simulink model "GasExample_V4"  (R2025b)
settings: Solver=FixedStepAuto  StartTime=0.0  StopTime=1000  FixedStep=0.01  RelTol=1e-3
libraries: Bibliothek_FHDO_V1 x22, simulink x8
settings Model: Creator=goessling  LastModifiedBy=goessling

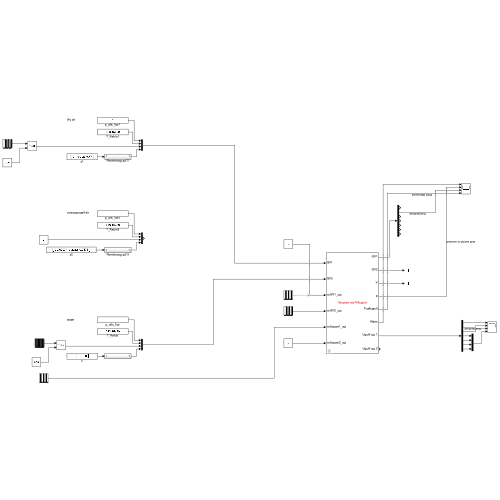
[thumbnail: Simulink's stored preview of the top-level diagram]
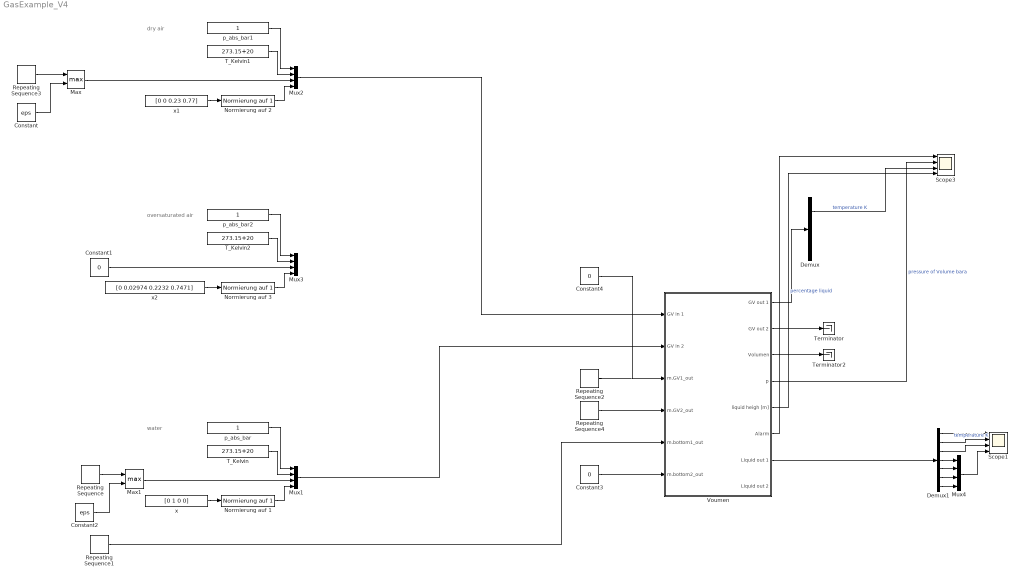
== system GasExample_V4 ==
  note: water
  note: dry air
  note: oversaturated air
  Constant : Constant  Value=eps
  Constant1 : Constant  Value=0
  Constant2 : Constant  Value=eps
  Constant3 : Constant  Value=0
  Constant4 : Constant  Value=0
  Demux : Demux  Outputs=7
  Demux1 : Demux  Outputs=7
  Max : MinMax  Function=max  Inputs=2
  Max1 : MinMax  Function=max  Inputs=2
  Mux{1..4} (4 alike) : Mux
  Normierung auf 1 : Bibliothek_FHDO_V1/Wasser/Normierung auf 1  SystemSampleTime=-1  VariantActivationTime=update diagram  EmptyChoice=off  PassThrough=off  PassThroughVariantControl=(default)  EmptyChoiceVariantControl=(default)  AllowFlexibleInterface=on  Latency=0  AutoFrameSizeCalculation=off
  Normierung auf 2 : Bibliothek_FHDO_V1/Wasser/Normierung auf 1  SystemSampleTime=-1  VariantActivationTime=update diagram  EmptyChoice=off  PassThrough=off  PassThroughVariantControl=(default)  EmptyChoiceVariantControl=(default)  AllowFlexibleInterface=on  Latency=0  AutoFrameSizeCalculation=off
  Normierung auf 3 : Bibliothek_FHDO_V1/Wasser/Normierung auf 1  SystemSampleTime=-1  VariantActivationTime=update diagram  EmptyChoice=off  PassThrough=off  PassThroughVariantControl=(default)  EmptyChoiceVariantControl=(default)  AllowFlexibleInterface=on  Latency=0  AutoFrameSizeCalculation=off
  Repeating Sequence : simulink/Sources/Repeating Sequence  rep_seq_t=[0 100 100.01 500 500.01 600 600.01 1000]  rep_seq_y=[1 1 0 0 1 1 0 0]*282.1778521
  Repeating Sequence1 : simulink/Sources/Repeating Sequence  rep_seq_t=[0 300 300.01 400 400.01 1000]  rep_seq_y=[0 0 1 1 0 0]*282.1778521
  Repeating Sequence2 : simulink/Sources/Repeating Sequence  rep_seq_t=[0 600 600.01 700 700.01 1000]  rep_seq_y=[0 0 1 1 0 0]*1
  Repeating Sequence3 : simulink/Sources/Repeating Sequence  rep_seq_t=[0 700 700.01 1000]  rep_seq_y=[0 0 1 1]*1
  Repeating Sequence4 : simulink/Sources/Repeating Sequence  rep_seq_t=[0 800 800.01 1000]  rep_seq_y=[0 0 1 1]*1
  Scope1 : Scope  NumInputPorts=4
      settings: ActiveDisplayYMinimum=0.9  ActiveDisplayYMaximum=1.1
  Scope3 : Scope  NumInputPorts=4
      settings: ActiveDisplayYMinimum=-0.12499999999999997  ActiveDisplayYMaximum=1.125
  T_Kelvin : Constant  Value=273.15+20
  T_Kelvin1 : Constant  Value=273.15+20
  T_Kelvin2 : Constant  Value=273.15+20
  Terminator : Terminator
  Terminator2 : Terminator
  Voumen : Subsystem  mask{A=70685.83471/1000000, h=0.8, p_start=1, T_start=20, x_start=[0 0.014732262 0.229444643 0.755823095], h_start=0}
      mask prompts: A "Area [m^2]"; h "heigh [m]"; p_start "p [bar]"; T_start "T [°C]"; x_start "x"; h_start "liquid level start [m]"
      mask Display:
      | color('red')
      | disp(['Volumen mit Füllstand'])
      | 
      | color('black')
      | port_label('input', 1, 'GV1')
      | port_label('input', 2, 'GV2')
      | port_label('input', 3, 'm.GV1_out')
      | port_label('input', 4, 'm.GV2_out')
      | port_label('input', 5, 'm.bottom1_out')
      | port_label('input', 6, 'm.bottom2_out')
      | 
      | 
      | port_label('output', 1, 'GV1')
      | port_label('output', 2, 'GV2')
      | port_label('output', 3, 'V')
      | port_label('output', 4, 'p')
      | port_label('output', 5, 'Fuellstand')
      | port_label('output', 6, 'Alarm')
      | port_label('output', 7, 'Liquid out 1')
      | port_label('output', 8, 'Liquid out 2')
  p_abs_bar : Constant
  p_abs_bar1 : Constant
  p_abs_bar2 : Constant
  x : Constant  Value=[0 1 0 0]
  x1 : Constant  Value=[0 0 0.23 0.77]
  x2 : Constant  Value=[0 0.02974 0.2232 0.7471]
  wires:
  Voumen/3(Volumen) -> Terminator2/1
  Voumen/4(p) -> Scope3/2  "pressure of Volume bara"
  Voumen/1(GV out 1) -> Demux/1
  Voumen/2(GV out 2) -> Terminator/1
  Demux/2 -> Scope3/3  "temperature K"
  Voumen/5(liquid heigh [m]) -> Scope3/4  "percentage liquid"
  x/1 -> Normierung auf 1/1
  p_abs_bar/1 -> Mux1/1
  Mux1/1 -> Voumen/2(GV in 2)
  Repeating Sequence/1 -> Max1/1
  Normierung auf 1/1 -> Mux1/4
  T_Kelvin/1 -> Mux1/2
  T_Kelvin1/1 -> Mux2/2
  Normierung auf 2/1 -> Mux2/4
  Repeating Sequence3/1 -> Max/1
  p_abs_bar1/1 -> Mux2/1
  x1/1 -> Normierung auf 2/1
  T_Kelvin2/1 -> Mux3/2
  p_abs_bar2/1 -> Mux3/1
  x2/1 -> Normierung auf 3/1
  Normierung auf 3/1 -> Mux3/4
  Constant1/1 -> Mux3/3
  Mux2/1 -> Voumen/1(GV in 1)
  Voumen/6(Alarm) -> Scope3/1
  Repeating Sequence1/1 -> Voumen/5(m.bottom1_out)
  Repeating Sequence4/1 -> Voumen/4(m.GV2_out)
  Constant3/1 -> Voumen/6(m.bottom2_out)
  Voumen/7(Liquid out 1) -> Demux1/1
  Demux1/1 -> Scope1/1
  Demux1/2 -> Scope1/2  "temperature K"
  Demux1/3 -> Scope1/3
  Demux1/4 -> Mux4/1
  Demux1/5 -> Mux4/2
  Demux1/6 -> Mux4/3
  Demux1/7 -> Mux4/4
  Mux4/1 -> Scope1/4
  Repeating Sequence2/1 -> ?
  Constant/1 -> Max/2
  Max/1 -> Mux2/3
  Constant2/1 -> Max1/2
  Max1/1 -> Mux1/3
  Constant4/1 -> Voumen/3(m.GV1_out)

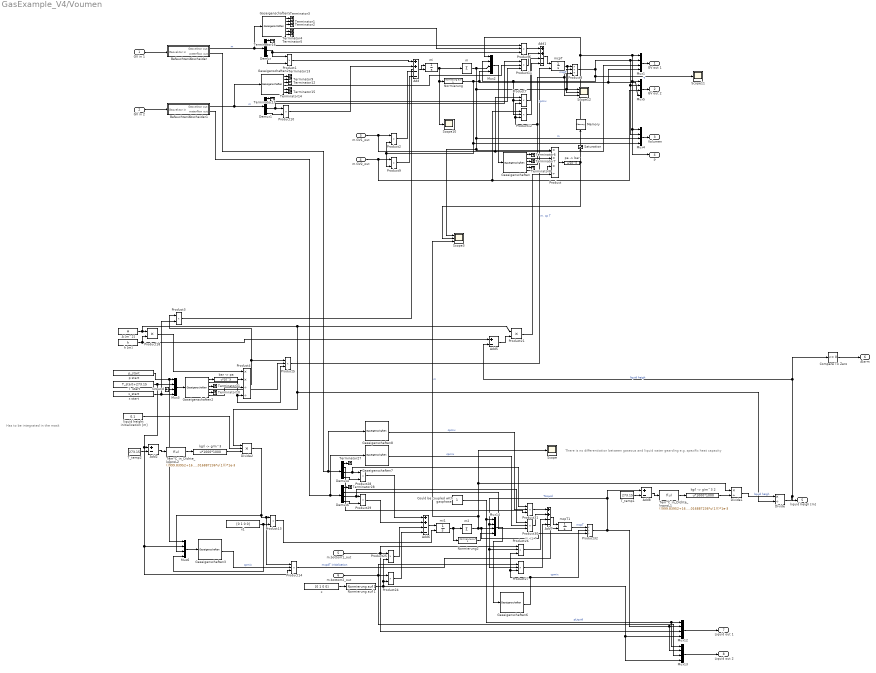
== system GasExample_V4/Voumen ==
  note: There is no differentiation between gaseous and liquid water gearding e.g. spezific heat capacity
  note: m. cp T
  note: Has to be integrated in the mask
  GV in 1 : Inport
  GV in 2 : Inport  Port=2
  m.GV1_out : Inport  Port=3
  m.GV2_out : Inport  Port=4
  m.bottom1_out : Inport  Port=5
  m.bottom2_out : Inport  Port=6
  A [m^2] : Constant  Value=A
  Add : Sum  Inputs=++--
  Add1 : Sum  Inputs=++--  SampleTime=.01
  Add2 : Sum  Inputs=+-
  Add5 : Sum  Inputs=+-
  Add6 : Sum  Inputs=++--
  Add7 : Sum  Inputs=++--  SampleTime=.01
  Add8 : Sum  Inputs=+-
  Befeuchter/Abscheider : Subsystem
      mask Display:
      | color('red')
      | disp('No Oversaturation');
      | 
      | color('black')
      | port_label('output', 1, 'GV')
      | port_label('output', 2, 'm.')
      | port_label('input', 1, 'GV')
  Befeuchter/Abscheider1 : Subsystem
      mask Display:
      | color('red')
      | disp('No Oversaturation');
      | 
      | color('black')
      | port_label('output', 1, 'GV')
      | port_label('output', 2, 'm.')
      | port_label('input', 1, 'GV')
  Compare To Zero : simulink/Logic and Bit Operations/Compare To Zero  relop=<=  OutDataTypeStr=boolean
  Could be coupled with gasphase : Constant
  Demux{,1,4,6} (4 alike) : Demux  Outputs=[1 1 1 4]
  Divide : Product  Inputs=*/
  Divide1 : Product  Inputs=*/
  Divide2 : Product  Inputs=3
  Gaseigenschaften{,1..3,5..8} (8 alike) : Bibliothek_FHDO_V1/Gaseigenschaften  SystemSampleTime=-1  VariantActivationTime=update diagram  EmptyChoice=off  PassThrough=off  PassThroughVariantControl=(default)  EmptyChoiceVariantControl=(default)  AllowFlexibleInterface=on  Latency=0  AutoFrameSizeCalculation=off
  Ground : Ground
  Memory : Memory  InitialCondition=p_start
  Mux{1..6,12..14} (9 alike) : Mux
  Normierung : Bibliothek_FHDO_V1/Sauerstoff/Normierung auf 1  SystemSampleTime=-1  VariantActivationTime=update diagram  EmptyChoice=off  PassThrough=off  PassThroughVariantControl=(default)  EmptyChoiceVariantControl=(default)  AllowFlexibleInterface=on  Latency=0  AutoFrameSizeCalculation=off
  Normierung auf 1 : Bibliothek_FHDO_V1/Wasser/Normierung auf 1  SystemSampleTime=-1  VariantActivationTime=update diagram  EmptyChoice=off  PassThrough=off  PassThroughVariantControl=(default)  EmptyChoiceVariantControl=(default)  AllowFlexibleInterface=on  Latency=0  AutoFrameSizeCalculation=off
  Normierung2 : Bibliothek_FHDO_V1/Sauerstoff/Normierung auf 1  SystemSampleTime=-1  VariantActivationTime=update diagram  EmptyChoice=off  PassThrough=off  PassThroughVariantControl=(default)  EmptyChoiceVariantControl=(default)  AllowFlexibleInterface=on  Latency=0  AutoFrameSizeCalculation=off
  Product : Product  Inputs=***/  RndMeth=Zero
  Product{1..3,9..10,13,24..25,28..29} (10 alike) : Product  RndMeth=Zero
  Product{5..7,11..12,14,26..27,30..31} (10 alike) : Product  Inputs=3  RndMeth=Zero
  Product18 : Product
  Product21 : Product
  Product32 : Product  Inputs=*//  RndMeth=Zero
  Product4 : Product  Inputs=**//  RndMeth=Zero
  Product8 : Product  Inputs=*//  RndMeth=Zero
  Saturation : Saturate  UpperLimit=inf  LowerLimit=1
  Scope : Scope
      settings: ActiveDisplayYMinimum=-2821.8113029993069  ActiveDisplayYMaximum=32452.183821075614  DataLoggingVariableName=ScopeData8
  Scope10 : Scope
      settings: ActiveDisplayYMinimum=-3527.53472  ActiveDisplayYMaximum=31747.81251  DataLoggingVariableName=ScopeData2
  Scope11 : Scope
      settings: ActiveDisplayYMinimum=289.4277  ActiveDisplayYMaximum=326.65069  DataLoggingVariableName=ScopeData3
  Scope12 : Scope  NumInputPorts=3
      settings: ActiveDisplayYMinimum=-1.92104645928E+6  ActiveDisplayYMaximum=1.750985915796E+7  DataLoggingVariableName=ScopeData4
  Scope3 : Scope  NumInputPorts=3
      settings: ActiveDisplayYMinimum=60.923032021236594  ActiveDisplayYMaximum=185.9230320213137
  T  start : Constant  Value=T_start+273.15
  T_temp1 : Constant  Value=273.15
  T_temp2 : Constant  Value=273.15
  Tem°C_in_Dichte_kgproL1 : Fcn  Expr=((999.83952+16.952577*u(1)-0.0079905127*u(1)^2-0.000046241757*u(1)^3+0.00000010584601*u(1)^4-0.00000000028103006*u(1)^5)/(1+0.016887236*u(1)))*1e-3
  Tem°C_in_Dichte_kgproL2 : Fcn  Expr=((999.83952+16.952577*u(1)-0.0079905127*u(1)^2-0.000046241757*u(1)^3+0.00000010584601*u(1)^4-0.00000000028103006*u(1)^5)/(1+0.016887236*u(1)))*1e-3
  Terminator{1..17,27..28} (19 alike) : Terminator
  "bar -> pa" : Fcn  Expr=u*10^5
  h [m] : Constant  Value=h
  "kg/l -> g/m^3" : Fcn  Expr=u*1000*1000
  "kg/l -> g/m^3 2" : Fcn  Expr=u*1000*1000
  liquid height initialization [m] : Constant  Value=0.1
  m : Sum  Inputs=+
  m2 : Sum  Inputs=+
  mcpT : Integrator  InitialConditionSource=external  InitialCondition=[0 0 0 0 0 0 .21 .79]*1293
  mcpT1 : Integrator  InitialConditionSource=external  InitialCondition=[0 0 0 0 0 0 .21 .79]*1293
  mi : Integrator  InitialConditionSource=external  InitialCondition=[0 0 0 0 0 0 .21 .79]*1293
  mi1 : Integrator  InitialConditionSource=external  InitialCondition=[0 0 0 0 0 0 .21 .79]*1293
  p start : Constant  Value=p_start
  "pa -> bar" : Fcn  Expr=u/10^5
  x : Constant  Value=[0 1 0 0]
  x start : Constant  Value=x_start
  x1 : Constant  Value=[0 1 0 0]
  GV out 1 : Outport
  GV out 2 : Outport  Port=2
  Volumen : Outport  Port=3
  p : Outport  Port=4
  liquid heigh [m] : Outport  Port=5
  Alarm : Outport  Port=6
  Liquid out 1 : Outport  Port=7
  Liquid out 2 : Outport  Port=8
  wires:
  GV in 1/1 -> Befeuchter/Abscheider/1(Gasvektor in)
  Demux/3 -> Product1/1, Product6/3
  Demux/2 -> Product6/1
  Demux/4 -> Product1/2
  Gaseigenschaften/1 -> Terminator6/1
  Gaseigenschaften/4 -> Product8/3, Scope12/3, Product7/3, Product12/3  "cpmix"
  Product1/1 -> Add/1
  m.GV1_out/1 -> Product2/1, Product7/1, Mux1/3
  Normierung/1 -> Mux2/4, Mux1/4, Mux5/4, Mux4/4, Product2/2, Product9/2
  Product2/1 -> Add/3
  Add/1 -> mi/1
  m/1 -> Mux2/3, Product8/2, Scope12/2, Scope3/1, Product/1, Mux4/3  "m"
  Gaseigenschaften5/1 -> Terminator3/1
  Gaseigenschaften5/4 -> Product6/2
  Gaseigenschaften/6 -> Product/3
  Gaseigenschaften/2 -> Product/2
  A [m^2]/1 -> Divide2/1, Divide/2, Product21/1, Product18/1
  Product/1 -> "pa -> bar"/1
  Mux1/1 -> GV out 1/1
  Gaseigenschaften5/2 -> Terminator1/1
  Gaseigenschaften5/3 -> Terminator2/1
  Gaseigenschaften5/5 -> Terminator4/1
  Gaseigenschaften5/6 -> Terminator5/1
  Gaseigenschaften/3 -> Terminator7/1
  Gaseigenschaften/5 -> Terminator8/1
  x start/1 -> Mux3/4, Product3/2
  Ground/1 -> Mux3/3
  p start/1 -> Mux6/1, Mux3/1
  T  start/1 -> Product14/3, Mux6/2, Add2/1, Mux3/2
  Mux3/1 -> Gaseigenschaften2/1
  Gaseigenschaften2/1 -> "bar -> pa"/1
  "bar -> pa"/1 -> Product4/2
  Gaseigenschaften2/6 -> Product4/3
  Gaseigenschaften2/2 -> Product4/4, Product5/3
  Gaseigenschaften2/3 -> Terminator11/1
  Gaseigenschaften2/4 -> Product5/2
  Gaseigenschaften2/5 -> Terminator10/1
  Product4/1 -> Product5/1, Product3/1
  Product3/1 -> mi/2
  Product5/1 -> mcpT/2  "m. cp T"
  Product6/1 -> Add1/1
  Add1/1 -> mcpT/1
  mcpT/1 -> Scope12/1, Product8/1  "mcpT"
  Product8/1 -> Mux2/2, Product7/2, Product12/2, Scope11/1, Mux1/2, Mux4/2, Mux5/2  "T"
  Product7/1 -> Add1/3
  m.GV2_out/1 -> Product9/1, Mux5/3, Product12/1
  Product9/1 -> Add/4
  Mux5/1 -> GV out 2/1
  Gaseigenschaften1/1 -> Terminator13/1
  Gaseigenschaften1/2 -> Terminator9/1
  Gaseigenschaften1/3 -> Terminator12/1
  Gaseigenschaften1/5 -> Terminator14/1
  Gaseigenschaften1/6 -> Terminator15/1
  Demux/1 -> Terminator16/1
  Demux1/1 -> Terminator17/1
  Demux1/3 -> Product10/1, Product11/3
  Demux1/4 -> Product10/2
  Product10/1 -> Add/2
  Product11/1 -> Add1/2
  Product12/1 -> Add1/4
  Gaseigenschaften1/4 -> Product11/2
  Demux1/2 -> Product11/1
  Saturation/1 -> Memory/1
  Mux4/1 -> Volumen/1
  mi/1 -> Scope10/1, Normierung/1, m/1
  h [m]/1 -> Add5/1, Product18/2
  Add5/1 -> Product21/2
  Product21/1 -> Product/4
  Product18/1 -> Product4/1
  "pa -> bar"/1 -> Saturation/1, Scope3/2
  Mux2/1 -> Gaseigenschaften/1
  x/1 -> Normierung auf 1/1
  Normierung auf 1/1 -> Mux13/4, Mux12/4, Product25/2, Product24/2
  m.bottom2_out/1 -> Product27/1, Mux13/3, Product24/1
  m.bottom1_out/1 -> Product26/1, Mux12/3, Product25/1
  Mux12/1 -> Liquid out 1/1
  Mux13/1 -> Liquid out 2/1
  Product25/1 -> Add6/3
  Product24/1 -> Add6/4
  Befeuchter/Abscheider/1(Gasvektor out) -> Gaseigenschaften5/1, Demux/1  "m"
  GV in 2/1 -> Befeuchter/Abscheider1/1(Gasvektor in)
  Befeuchter/Abscheider1/1(Gasvektor out) -> Gaseigenschaften1/1, Demux1/1  "m"
  Befeuchter/Abscheider/2(waterflow out) -> Gaseigenschaften8/1, Demux4/1
  Befeuchter/Abscheider1/2(waterflow out) -> Gaseigenschaften7/1, Demux6/1
  Demux4/4 -> Product28/2
  Demux4/1 -> Terminator27/1
  Demux4/3 -> Product31/1, Product28/1
  Demux6/3 -> Product30/1, Product29/1
  Demux6/1 -> Terminator28/1
  Demux6/4 -> Product29/2
  Product28/1 -> Add6/1
  Product29/1 -> Add6/2
  Add6/1 -> mi1/1
  mi1/1 -> Normierung2/1, m2/1
  m2/1 -> Scope3/3, Scope/1, Divide1/1, Product32/3, Mux14/3  "m"
  Could be coupled with gasphase/1 -> Mux13/1, Mux12/1, Mux14/1  "pLiquid"
  Product32/1 -> Mux13/2, Mux12/2, Add8/1, Product27/2, Product26/2, Mux14/2  "TLiquid"
  Normierung2/1 -> Mux14/4
  Mux14/1 -> Gaseigenschaften6/1
  Gaseigenschaften8/4 -> Product31/2  "cpmix"
  Gaseigenschaften7/4 -> Product30/2  "cpmix"
  Demux4/2 -> Product31/3
  Demux6/2 -> Product30/3
  Product31/1 -> Add7/1
  Product30/1 -> Add7/2
  Gaseigenschaften6/4 -> Product32/2, Product27/3, Product26/3  "cpmix"
  Product26/1 -> Add7/3
  Product27/1 -> Add7/4
  Add7/1 -> mcpT1/1
  mcpT1/1 -> Product32/1  "mcpT"
  Tem°C_in_Dichte_kgproL1/1 -> "kg/l -> g/m^3 2"/1
  T_temp1/1 -> Add8/2
  Add8/1 -> Tem°C_in_Dichte_kgproL1/1
  "kg/l -> g/m^3 2"/1 -> Divide1/2
  Divide/1 -> Add5/2, Compare To Zero/1, liquid heigh [m]/1  "liquid heigh"
  Divide1/1 -> Divide/1  "liquid heigh"
  Divide2/1 -> Mux6/3, Product14/1, Product13/1
  Memory/1 -> Mux2/1, Mux1/1, Mux5/1, Mux4/1, p/1
  Compare To Zero/1 -> Alarm/1
  "kg/l -> g/m^3"/1 -> Divide2/3
  Add2/1 -> Tem°C_in_Dichte_kgproL2/1
  T_temp2/1 -> Add2/2
  Tem°C_in_Dichte_kgproL2/1 -> "kg/l -> g/m^3"/1
  liquid height initialization [m]/1 -> Divide2/2
  x1/1 -> Product13/2, Mux6/4
  Product13/1 -> mi1/2
  Mux6/1 -> Gaseigenschaften3/1
  Gaseigenschaften3/4 -> Product14/2  "cpmix"
  Product14/1 -> mcpT1/2  "mcpdT initialization"

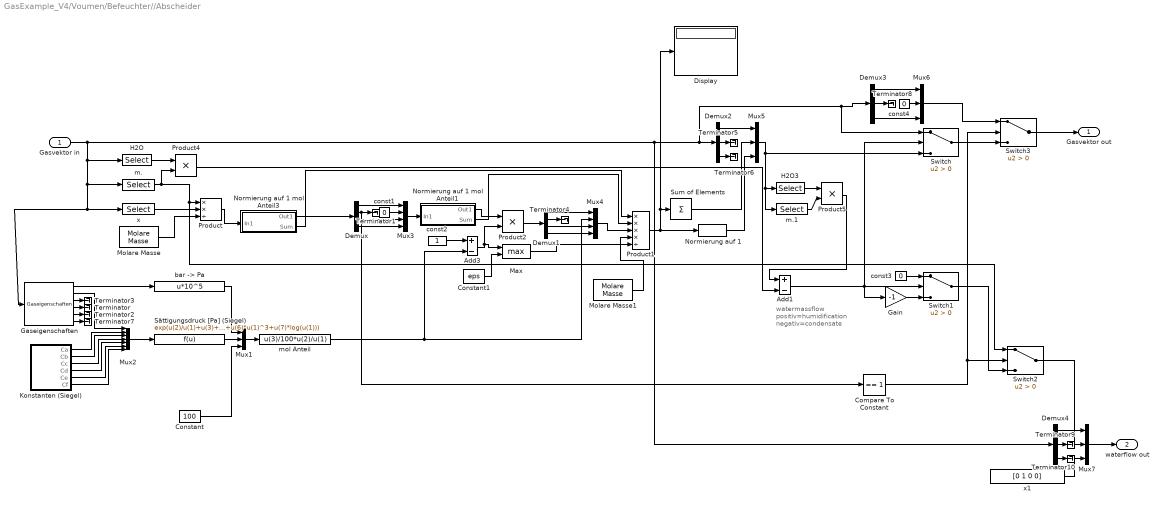
== system GasExample_V4/Voumen/Befeuchter//Abscheider ==
  note: watermassflow
      | positiv=humidification
      | negativ=condensate
  Gasvektor in : Inport
  Add1 : Sum  Inputs=+-
  Add3 : Sum  Inputs=+-
  Compare To Constant : simulink/Logic and Bit Operations/Compare To Constant  relop===  const=1  OutDataTypeStr=boolean
  Constant : Constant  Value=100
  Constant1 : Constant  Value=eps
  Demux : Demux
  Demux1 : Demux
  Demux2 : Demux  Outputs=[2 1 4]
  Demux3 : Demux  Outputs=[2 1 4]
  Demux4 : Demux  Outputs=[2 1 4]
  Display : Display
  Gain : Gain  Gain=-1
  Gaseigenschaften : Bibliothek_FHDO_V1/Gaseigenschaften  SystemSampleTime=-1  VariantActivationTime=update diagram  EmptyChoice=off  PassThrough=off  PassThroughVariantControl=(default)  EmptyChoiceVariantControl=(default)  AllowFlexibleInterface=on  Latency=0  AutoFrameSizeCalculation=off
  H2O : Selector  InputPortWidth=7  IndexOptions=Index vector (dialog)  Indices=5  OutputSizes=1
  H2O3 : Selector  InputPortWidth=7  IndexOptions=Index vector (dialog)  Indices=5  OutputSizes=1
  Konstanten (Siegel) : Subsystem
  Max : MinMax  Function=max  Inputs=2
  Molare Masse : Bibliothek_FHDO_V1/Molare Masse  SystemSampleTime=-1  VariantActivationTime=update diagram  EmptyChoice=off  PassThrough=off  PassThroughVariantControl=(default)  EmptyChoiceVariantControl=(default)  AllowFlexibleInterface=on  Latency=0  AutoFrameSizeCalculation=off
  Molare Masse1 : Bibliothek_FHDO_V1/Molare Masse  SystemSampleTime=-1  VariantActivationTime=update diagram  EmptyChoice=off  PassThrough=off  PassThroughVariantControl=(default)  EmptyChoiceVariantControl=(default)  AllowFlexibleInterface=on  Latency=0  AutoFrameSizeCalculation=off
  Mux{1,5..7} (4 alike) : Mux  Inputs=3
  Mux2 : Mux  Inputs=7
  Mux3 : Mux
  Mux4 : Mux
  Normierung auf 1 : Bibliothek_FHDO_V1/Sauerstoff/Normierung auf 1  SystemSampleTime=-1  VariantActivationTime=update diagram  EmptyChoice=off  PassThrough=off  PassThroughVariantControl=(default)  EmptyChoiceVariantControl=(default)  AllowFlexibleInterface=on  Latency=0  AutoFrameSizeCalculation=off
  Normierung auf 1 mol Anteil1 : Subsystem
  Normierung auf 1 mol Anteil3 : Subsystem
  Product : Product  Inputs=**/  RndMeth=Zero
  Product1 : Product  Inputs=****/  RndMeth=Zero
  Product2 : Product  RndMeth=Zero
  Product4 : Product  RndMeth=Zero
  Product5 : Product  RndMeth=Zero
  Sum of Elements : Sum  Inputs=+
  Switch{,1..3} (4 alike) : Switch  Criteria=u2 > Threshold  SaturateOnIntegerOverflow=off  InputSameDT=off
  Sättigungsdruck [Pa] (Siegel) : Fcn  Expr=exp(u(2)/u(1)+u(3)+u(4)*u(1)+u(5)*u(1)^2+u(6)*u(1)^3+u(7)*log(u(1)))
  Terminator{,1..10} (11 alike) : Terminator
  "bar -> Pa" : Fcn  Expr=u*10^5
  const1 : Constant  Value=0
  const2 : Constant
  const3 : Constant  Value=0
  const4 : Constant  Value=0
  m. : Selector  InputPortWidth=7  IndexOptions=Index vector (dialog)  Indices=3  OutputSizes=1
  m.1 : Selector  InputPortWidth=7  IndexOptions=Index vector (dialog)  Indices=3  OutputSizes=1
  mol Anteil : Fcn  Expr=u(3)/100*u(2)/u(1)
  x : Selector  InputPortWidth=7  IndexOptions=Index vector (dialog)  Indices=[4 5 6 7]  OutputSizes=1
  x1 : Constant  Value=[0 1 0 0]
  Gasvektor out : Outport
  waterflow out : Outport  Port=2
  wires:
  Demux1/4 -> Mux4/4
  Demux1/3 -> Mux4/3
  Demux1/1 -> Mux4/1
  Demux1/2 -> Terminator4/1
  Demux/4 -> Mux3/4
  Demux/3 -> Mux3/3
  Demux/1 -> Mux3/1
  const1/1 -> Mux3/2
  Demux/2 -> Compare To Constant/1, Terminator1/1
  Product4/1 -> Add1/2
  Product5/1 -> Add1/1
  H2O3/1 -> Product5/1
  m.1/1 -> Product5/2
  H2O/1 -> Product4/1
  Normierung auf 1 mol Anteil1/2(Sum) -> Product1/2
  Normierung auf 1 mol Anteil3/2(Sum) -> Product1/1
  Normierung auf 1 mol Anteil3/1(Out1) -> Demux/1
  Normierung auf 1/1 -> Mux5/3
  Mux5/1 -> Switch/3, m.1/1, H2O3/1
  Demux2/3 -> Terminator6/1
  Demux2/2 -> Terminator5/1
  Product1/1 -> Normierung auf 1/1, Display/1, Sum of Elements/1
  Sum of Elements/1 -> Mux5/2
  Demux2/1 -> Mux5/1
  m./1 -> Switch2/1, Product/1, Product4/2
  Molare Masse1/1 -> Product1/4
  Mux4/1 -> Product1/3
  Product2/1 -> Demux1/1
  Add3/1 -> Max/1, Product2/2
  Normierung auf 1 mol Anteil1/1(Out1) -> Product2/1
  mol Anteil/1 -> Mux4/2, Add3/2
  const2/1 -> Add3/1
  Mux3/1 -> Normierung auf 1 mol Anteil1/1(In1)
  Product/1 -> Normierung auf 1 mol Anteil3/1(In1)
  Molare Masse/1 -> Product/3
  x/1 -> Product/2
  "bar -> Pa"/1 -> Mux1/1
  Constant/1 -> Mux1/3
  Mux1/1 -> mol Anteil/1
  Sättigungsdruck [Pa] (Siegel)/1 -> Mux1/2
  Mux2/1 -> Sättigungsdruck [Pa] (Siegel)/1
  Gaseigenschaften/5 -> Terminator2/1
  Gaseigenschaften/4 -> Terminator/1
  Gaseigenschaften/3 -> Terminator3/1
  Gaseigenschaften/1 -> "bar -> Pa"/1
  Konstanten (Siegel)/6(Cf) -> Mux2/7
  Konstanten (Siegel)/5(Ce) -> Mux2/6
  Konstanten (Siegel)/4(Cd) -> Mux2/5
  Konstanten (Siegel)/3(Cc) -> Mux2/4
  Konstanten (Siegel)/2(Cb) -> Mux2/3
  Konstanten (Siegel)/1(Ca) -> Mux2/2
  Gaseigenschaften/2 -> Mux2/1
  Gasvektor in/1 -> Demux3/1, Switch/1, Demux2/1, Demux4/1, H2O/1, Gaseigenschaften/1, x/1, m./1
  Gaseigenschaften/6 -> Terminator7/1
  Add1/1 -> Gain/1, Switch1/2, Switch/2
  Switch/1 -> Switch3/3
  const3/1 -> Switch1/1
  Compare To Constant/1 -> Switch3/2, Switch2/2
  Switch2/1 -> Mux7/2
  Switch1/1 -> Switch2/3
  Demux3/1 -> Mux6/1
  Demux3/3 -> Mux6/3
  const4/1 -> Mux6/2
  Demux3/2 -> Terminator8/1
  Mux6/1 -> Switch3/1
  Switch3/1 -> Gasvektor out/1
  Demux4/1 -> Mux7/1
  Demux4/2 -> Terminator9/1
  Demux4/3 -> Terminator10/1
  x1/1 -> Mux7/3
  Mux7/1 -> waterflow out/1
  Gain/1 -> Switch1/3
  Constant1/1 -> Max/2
  Max/1 -> Product1/5

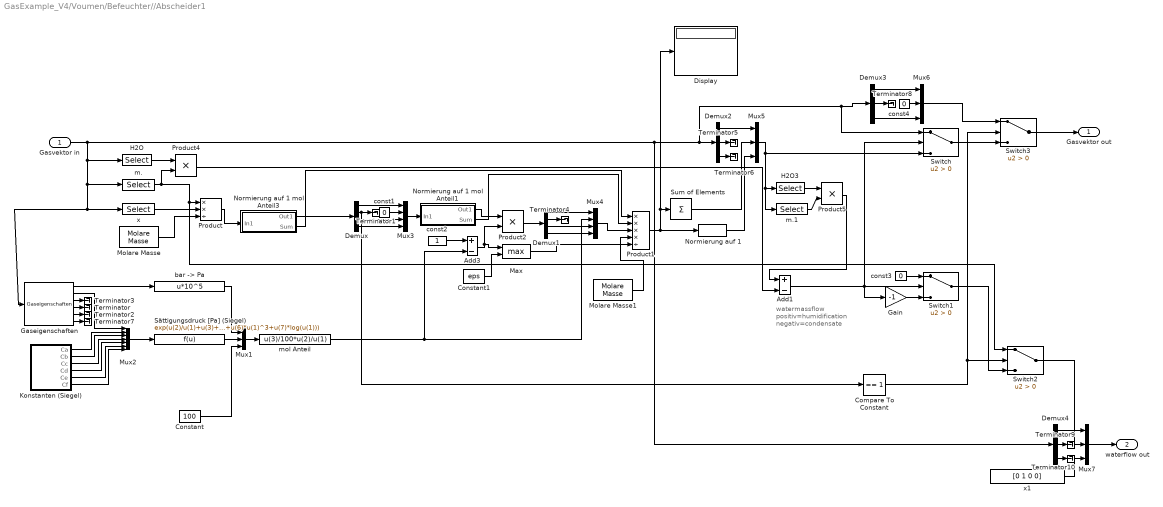
== system GasExample_V4/Voumen/Befeuchter//Abscheider1 ==
  note: watermassflow
      | positiv=humidification
      | negativ=condensate
  Gasvektor in : Inport
  Add1 : Sum  Inputs=+-
  Add3 : Sum  Inputs=+-
  Compare To Constant : simulink/Logic and Bit Operations/Compare To Constant  relop===  const=1  OutDataTypeStr=boolean
  Constant : Constant  Value=100
  Constant1 : Constant  Value=eps
  Demux : Demux
  Demux1 : Demux
  Demux2 : Demux  Outputs=[2 1 4]
  Demux3 : Demux  Outputs=[2 1 4]
  Demux4 : Demux  Outputs=[2 1 4]
  Display : Display
  Gain : Gain  Gain=-1
  Gaseigenschaften : Bibliothek_FHDO_V1/Gaseigenschaften  SystemSampleTime=-1  VariantActivationTime=update diagram  EmptyChoice=off  PassThrough=off  PassThroughVariantControl=(default)  EmptyChoiceVariantControl=(default)  AllowFlexibleInterface=on  Latency=0  AutoFrameSizeCalculation=off
  H2O : Selector  InputPortWidth=7  IndexOptions=Index vector (dialog)  Indices=5  OutputSizes=1
  H2O3 : Selector  InputPortWidth=7  IndexOptions=Index vector (dialog)  Indices=5  OutputSizes=1
  Konstanten (Siegel) : Subsystem
  Max : MinMax  Function=max  Inputs=2
  Molare Masse : Bibliothek_FHDO_V1/Molare Masse  SystemSampleTime=-1  VariantActivationTime=update diagram  EmptyChoice=off  PassThrough=off  PassThroughVariantControl=(default)  EmptyChoiceVariantControl=(default)  AllowFlexibleInterface=on  Latency=0  AutoFrameSizeCalculation=off
  Molare Masse1 : Bibliothek_FHDO_V1/Molare Masse  SystemSampleTime=-1  VariantActivationTime=update diagram  EmptyChoice=off  PassThrough=off  PassThroughVariantControl=(default)  EmptyChoiceVariantControl=(default)  AllowFlexibleInterface=on  Latency=0  AutoFrameSizeCalculation=off
  Mux{1,5..7} (4 alike) : Mux  Inputs=3
  Mux2 : Mux  Inputs=7
  Mux3 : Mux
  Mux4 : Mux
  Normierung auf 1 : Bibliothek_FHDO_V1/Sauerstoff/Normierung auf 1  SystemSampleTime=-1  VariantActivationTime=update diagram  EmptyChoice=off  PassThrough=off  PassThroughVariantControl=(default)  EmptyChoiceVariantControl=(default)  AllowFlexibleInterface=on  Latency=0  AutoFrameSizeCalculation=off
  Normierung auf 1 mol Anteil1 : Subsystem
  Normierung auf 1 mol Anteil3 : Subsystem
  Product : Product  Inputs=**/  RndMeth=Zero
  Product1 : Product  Inputs=****/  RndMeth=Zero
  Product2 : Product  RndMeth=Zero
  Product4 : Product  RndMeth=Zero
  Product5 : Product  RndMeth=Zero
  Sum of Elements : Sum  Inputs=+
  Switch{,1..3} (4 alike) : Switch  Criteria=u2 > Threshold  SaturateOnIntegerOverflow=off  InputSameDT=off
  Sättigungsdruck [Pa] (Siegel) : Fcn  Expr=exp(u(2)/u(1)+u(3)+u(4)*u(1)+u(5)*u(1)^2+u(6)*u(1)^3+u(7)*log(u(1)))
  Terminator{,1..10} (11 alike) : Terminator
  "bar -> Pa" : Fcn  Expr=u*10^5
  const1 : Constant  Value=0
  const2 : Constant
  const3 : Constant  Value=0
  const4 : Constant  Value=0
  m. : Selector  InputPortWidth=7  IndexOptions=Index vector (dialog)  Indices=3  OutputSizes=1
  m.1 : Selector  InputPortWidth=7  IndexOptions=Index vector (dialog)  Indices=3  OutputSizes=1
  mol Anteil : Fcn  Expr=u(3)/100*u(2)/u(1)
  x : Selector  InputPortWidth=7  IndexOptions=Index vector (dialog)  Indices=[4 5 6 7]  OutputSizes=1
  x1 : Constant  Value=[0 1 0 0]
  Gasvektor out : Outport
  waterflow out : Outport  Port=2
  wires:
  Max/1 -> Product1/5
  Constant1/1 -> Max/2
  Gain/1 -> Switch1/3
  Mux7/1 -> waterflow out/1
  x1/1 -> Mux7/3
  Demux4/3 -> Terminator10/1
  Demux4/2 -> Terminator9/1
  Demux4/1 -> Mux7/1
  Switch3/1 -> Gasvektor out/1
  Mux6/1 -> Switch3/1
  Demux3/2 -> Terminator8/1
  const4/1 -> Mux6/2
  Demux3/3 -> Mux6/3
  Demux3/1 -> Mux6/1
  Switch1/1 -> Switch2/3
  Switch2/1 -> Mux7/2
  Compare To Constant/1 -> Switch2/2, Switch3/2
  const3/1 -> Switch1/1
  Switch/1 -> Switch3/3
  Add1/1 -> Switch/2, Switch1/2, Gain/1
  Gaseigenschaften/6 -> Terminator7/1
  Gasvektor in/1 -> m./1, x/1, Gaseigenschaften/1, H2O/1, Demux4/1, Demux2/1, Switch/1, Demux3/1
  Gaseigenschaften/2 -> Mux2/1
  Konstanten (Siegel)/1(Ca) -> Mux2/2
  Konstanten (Siegel)/2(Cb) -> Mux2/3
  Konstanten (Siegel)/3(Cc) -> Mux2/4
  Konstanten (Siegel)/4(Cd) -> Mux2/5
  Konstanten (Siegel)/5(Ce) -> Mux2/6
  Konstanten (Siegel)/6(Cf) -> Mux2/7
  Gaseigenschaften/1 -> "bar -> Pa"/1
  Gaseigenschaften/3 -> Terminator3/1
  Gaseigenschaften/4 -> Terminator/1
  Gaseigenschaften/5 -> Terminator2/1
  Mux2/1 -> Sättigungsdruck [Pa] (Siegel)/1
  Sättigungsdruck [Pa] (Siegel)/1 -> Mux1/2
  Mux1/1 -> mol Anteil/1
  Constant/1 -> Mux1/3
  "bar -> Pa"/1 -> Mux1/1
  x/1 -> Product/2
  Molare Masse/1 -> Product/3
  Product/1 -> Normierung auf 1 mol Anteil3/1(In1)
  Mux3/1 -> Normierung auf 1 mol Anteil1/1(In1)
  const2/1 -> Add3/1
  mol Anteil/1 -> Add3/2, Mux4/2
  Normierung auf 1 mol Anteil1/1(Out1) -> Product2/1
  Add3/1 -> Product2/2, Max/1
  Product2/1 -> Demux1/1
  Mux4/1 -> Product1/3
  Molare Masse1/1 -> Product1/4
  m./1 -> Product4/2, Product/1, Switch2/1
  Demux2/1 -> Mux5/1
  Sum of Elements/1 -> Mux5/2
  Product1/1 -> Sum of Elements/1, Display/1, Normierung auf 1/1
  Demux2/2 -> Terminator5/1
  Demux2/3 -> Terminator6/1
  Mux5/1 -> H2O3/1, m.1/1, Switch/3
  Normierung auf 1/1 -> Mux5/3
  Normierung auf 1 mol Anteil3/1(Out1) -> Demux/1
  Normierung auf 1 mol Anteil3/2(Sum) -> Product1/1
  Normierung auf 1 mol Anteil1/2(Sum) -> Product1/2
  H2O/1 -> Product4/1
  m.1/1 -> Product5/2
  H2O3/1 -> Product5/1
  Product5/1 -> Add1/1
  Product4/1 -> Add1/2
  Demux/2 -> Terminator1/1, Compare To Constant/1
  const1/1 -> Mux3/2
  Demux/1 -> Mux3/1
  Demux/3 -> Mux3/3
  Demux/4 -> Mux3/4
  Demux1/2 -> Terminator4/1
  Demux1/1 -> Mux4/1
  Demux1/3 -> Mux4/3
  Demux1/4 -> Mux4/4

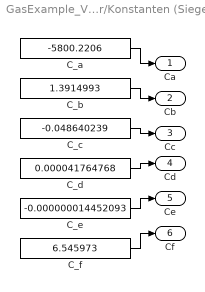
== system GasExample_V4/Voumen/Befeuchter//Abscheider/Konstanten (Siegel) ==
  C_a : Constant  Value=-5800.2206
  C_b : Constant  Value=1.3914993
  C_c : Constant  Value=-0.048640239
  C_d : Constant  Value=0.000041764768
  C_e : Constant  Value=-0.000000014452093
  C_f : Constant  Value=6.545973
  Ca : Outport
  Cb : Outport  Port=2
  Cc : Outport  Port=3
  Cd : Outport  Port=4
  Ce : Outport  Port=5
  Cf : Outport  Port=6
  wires:
  C_f/1 -> Cf/1
  C_e/1 -> Ce/1
  C_d/1 -> Cd/1
  C_c/1 -> Cc/1
  C_b/1 -> Cb/1
  C_a/1 -> Ca/1

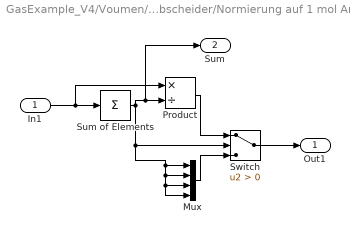
== system GasExample_V4/Voumen/Befeuchter//Abscheider/Normierung auf 1 mol Anteil1 ==
  In1 : Inport
  Mux : Mux
  Product : Product  Inputs=*/  RndMeth=Zero
  Sum of Elements : Sum  Inputs=+
  Switch : Switch  Criteria=u2 > Threshold  SaturateOnIntegerOverflow=off  InputSameDT=off
  Out1 : Outport
  Sum : Outport  Port=2
  wires:
  In1/1 -> Sum of Elements/1, Product/1
  Sum of Elements/1 -> Switch/2, Mux/4, Mux/3, Mux/2, Mux/1, Product/2, Sum/1
  Product/1 -> Switch/1
  Switch/1 -> Out1/1
  Mux/1 -> Switch/3

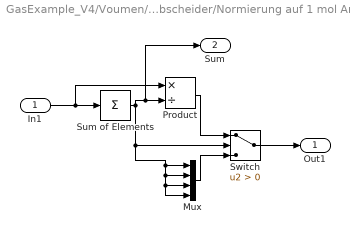
== system GasExample_V4/Voumen/Befeuchter//Abscheider/Normierung auf 1 mol Anteil3 ==
  In1 : Inport
  Mux : Mux
  Product : Product  Inputs=*/  RndMeth=Zero
  Sum of Elements : Sum  Inputs=+
  Switch : Switch  Criteria=u2 > Threshold  SaturateOnIntegerOverflow=off  InputSameDT=off
  Out1 : Outport
  Sum : Outport  Port=2
  wires:
  Mux/1 -> Switch/3
  Switch/1 -> Out1/1
  Product/1 -> Switch/1
  Sum of Elements/1 -> Sum/1, Product/2, Mux/1, Mux/2, Mux/3, Mux/4, Switch/2
  In1/1 -> Product/1, Sum of Elements/1

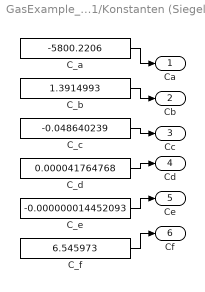
== system GasExample_V4/Voumen/Befeuchter//Abscheider1/Konstanten (Siegel) ==
  C_a : Constant  Value=-5800.2206
  C_b : Constant  Value=1.3914993
  C_c : Constant  Value=-0.048640239
  C_d : Constant  Value=0.000041764768
  C_e : Constant  Value=-0.000000014452093
  C_f : Constant  Value=6.545973
  Ca : Outport
  Cb : Outport  Port=2
  Cc : Outport  Port=3
  Cd : Outport  Port=4
  Ce : Outport  Port=5
  Cf : Outport  Port=6
  wires:
  C_a/1 -> Ca/1
  C_b/1 -> Cb/1
  C_c/1 -> Cc/1
  C_d/1 -> Cd/1
  C_e/1 -> Ce/1
  C_f/1 -> Cf/1

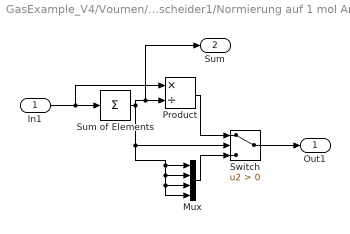
== system GasExample_V4/Voumen/Befeuchter//Abscheider1/Normierung auf 1 mol Anteil1 ==
  In1 : Inport
  Mux : Mux
  Product : Product  Inputs=*/  RndMeth=Zero
  Sum of Elements : Sum  Inputs=+
  Switch : Switch  Criteria=u2 > Threshold  SaturateOnIntegerOverflow=off  InputSameDT=off
  Out1 : Outport
  Sum : Outport  Port=2
  wires:
  Mux/1 -> Switch/3
  Switch/1 -> Out1/1
  Product/1 -> Switch/1
  Sum of Elements/1 -> Sum/1, Product/2, Mux/1, Mux/2, Mux/3, Mux/4, Switch/2
  In1/1 -> Product/1, Sum of Elements/1

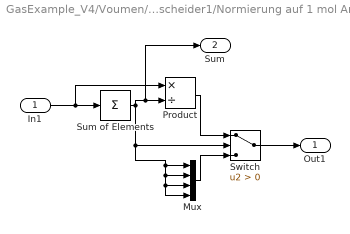
== system GasExample_V4/Voumen/Befeuchter//Abscheider1/Normierung auf 1 mol Anteil3 ==
  In1 : Inport
  Mux : Mux
  Product : Product  Inputs=*/  RndMeth=Zero
  Sum of Elements : Sum  Inputs=+
  Switch : Switch  Criteria=u2 > Threshold  SaturateOnIntegerOverflow=off  InputSameDT=off
  Out1 : Outport
  Sum : Outport  Port=2
  wires:
  In1/1 -> Sum of Elements/1, Product/1
  Sum of Elements/1 -> Switch/2, Mux/4, Mux/3, Mux/2, Mux/1, Product/2, Sum/1
  Product/1 -> Switch/1
  Switch/1 -> Out1/1
  Mux/1 -> Switch/3
